simulink model "kinovaMicoSimscapeModel"  (R2021b)
settings: Solver=VariableStepAuto  StartTime=0.0  StopTime=0.3  FixedStep=0.01  RelTol=1e-3
PostLoadFcn:
  | micoRigidBodyTreeCreation;
  | IC=deg2rad([-90,180,180,0,0,0]);
  | interactiveHomePosition=deg2rad([-90 90 177.5 90 0 0]');
  | load("./KinovaMicoSimscapeVariantConfigurations.mat");
values from neighbouring files (symbols this model uses):
  micoCandlePosition = deg2rad([0,180,180,0,0,0])    [KinovaMicoSimscapeInitializeScript.m]    (also in generatingRandomTrajectory.m)
  ViaPointsTaskSpace = [ViaPointsTaskSpace;[[pi;0;pi],[pi;0;pi],[pi;0;pi],[pi;0;pi],[0;0;0],[0;0;0],[pi;0;pi]]]    [KinovaMicoSimscapeInitializeScript.m]    (also in generatingRandomTrajectory.m = [ViaPointsTaskSpace;zeros(3,7)])
undefined symbols (not defined in the file or in its folder): Mico, ViaPointsJointSpace, X, Y, Z
libraries: sm_lib x26, nesl_utility x19, robotcorelib x4, robotmaniplib x3, pid_lib x2
(part 1 of 50)
settings Model: VariantConfigurationObject=KinovaMicoSimscapeVariantConfigurations  Creator=Chris  LastModifiedBy=morle
settings SolverCC: AlgebraicLoopSolver=TrustRegion
settings DebuggingCC: SFMachineParentedDataDiag=warning

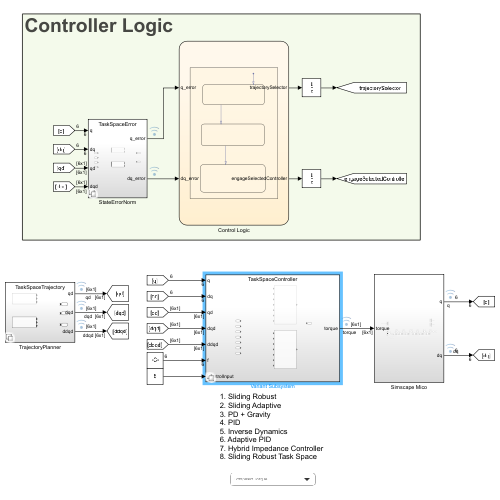
[thumbnail: Simulink's stored preview of the top-level diagram]
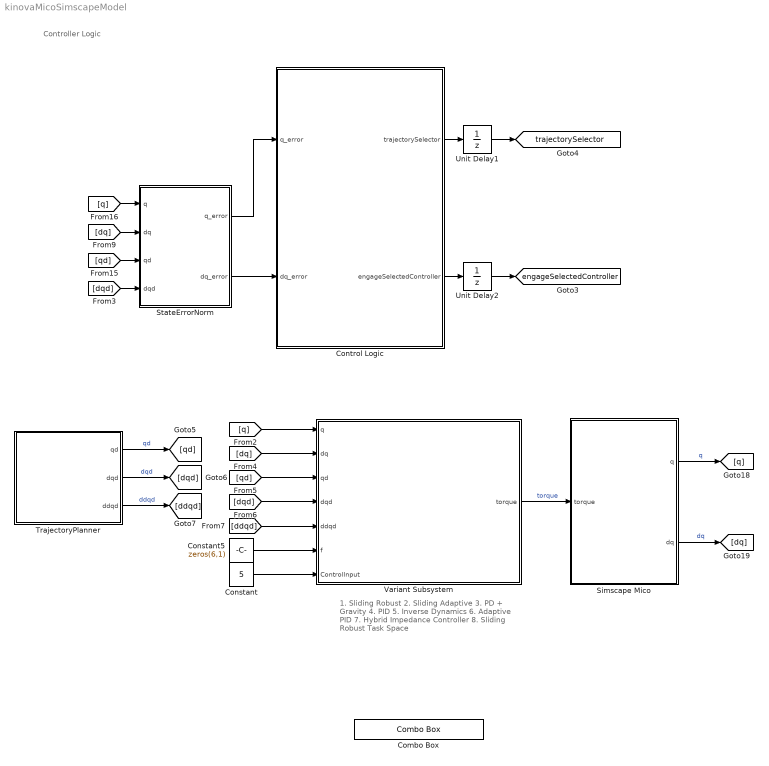
== system kinovaMicoSimscapeModel ==
  note: 1. Sliding Robust
      | 2. Sliding Adaptive
      | 3. PD + Gravity
      | 4. PID
      | 5. Inverse Dynamics
      | 6. Adaptive PID
      | 7. Hybrid Impedance Controller
      | 8. Sliding Robust Task Space
  note: Controller Logic
  Combo Box : ComboBox  LabelPosition=Hide  SelectedLabel=Computed Torque
      settings: Values={{'Sliding Robust Control', 'Sliding Adaptive Control', 'PD + Gravity', 'PID', 'Computed Torque', 'Adaptive PID', 'Hybrid Impedance Control', 'Sliding Robust Task Space'}, [1 2 3 4 5 6 7 8]}
  Constant : Constant  Value=5
  Constant5 : Constant  Value=zeros(6,1)
  Control Logic : Stateflow chart  TreatAsAtomicUnit=on
  Simscape Mico : Subsystem
  StateErrorNorm : Subsystem  Variant=on
  TrajectoryPlanner : Subsystem  Variant=on
  Unit Delay1 : UnitDelay  SampleTime=-1  HasFrameUpgradeWarning=on
  Unit Delay2 : UnitDelay  SampleTime=-1  HasFrameUpgradeWarning=on
  Variant Subsystem : Subsystem  Variant=on
  tag scope: engageSelectedController=global, trajectorySelector=global
  wires:
  Control Logic/2(engageSelectedController) -> Unit Delay2/1
  Unit Delay2/1 -> [engageSelectedController]
  Simscape Mico/2(dq) -> [dq]  "dq"
  Simscape Mico/1(q) -> [q]  "q"
  [dqd] -> Variant Subsystem/4(dqd)
  [ddqd] -> Variant Subsystem/5(ddqd)
  Constant5/1 -> Variant Subsystem/6(f)
  [dqd] -> StateErrorNorm/4(dqd)
  [dq] -> StateErrorNorm/2(dq)
  [qd] -> StateErrorNorm/3(qd)
  [q] -> StateErrorNorm/1(q)
  Variant Subsystem/1(torque) -> Simscape Mico/1(torque)  "torque"
  Unit Delay1/1 -> [trajectorySelector]
  Control Logic/1(trajectorySelector) -> Unit Delay1/1
  Constant/1 -> Variant Subsystem/7(ControlInput)
  [q] -> Variant Subsystem/1(q)
  [dq] -> Variant Subsystem/2(dq)
  [qd] -> Variant Subsystem/3(qd)
  StateErrorNorm/2(dq_error) -> Control Logic/2(dq_error)
  StateErrorNorm/1(q_error) -> Control Logic/1(q_error)
  TrajectoryPlanner/2(dqd) -> [dqd]  "dqd"
  TrajectoryPlanner/1(qd) -> [qd]  "qd"
  TrajectoryPlanner/3(ddqd) -> [ddqd]  "ddqd"

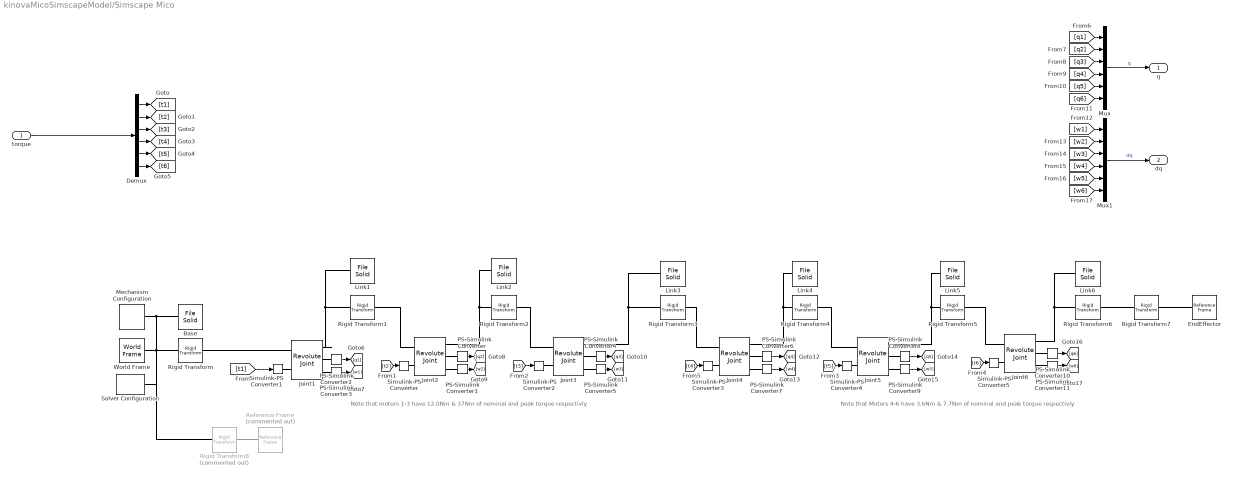
== system kinovaMicoSimscapeModel/Simscape Mico ==
  note: Note that motors 1-3 have 12.0Nm & 37Nm of nominal and peak torque respectivly
  note: Note that Motors 4-6 have 3.6Nm & 7.7Nm of nominal and peak torque respectivly
  torque : Inport
  Base : sm_lib/Body Elements/File Solid  ExtGeomFileName=.\StepFiles\Base.step  UnitType=FromFile  ExtGeomFileUnits=m  StepReaderType=HEX  ExportConvexHullGeometry=off  InertiaType=Custom  Mass=0  MassUnits=kg  CenterOfMass=[0 0 0]  CenterOfMassUnits=m  MomentsOfInertia=[0 0 0]  MomentsOfInertiaUnits=kg*m^2  ProductsOfInertia=[0 0 0]  ProductsOfInertiaUnits=kg*m^2  BasedOnType=Density  Density=1000  DensityUnits=kg/m^3  DoExposeReferenceFrame=on  SerializedFrames=<Frames/>  GraphicType=FromGeometry  MarkerShape=Sphere  MarkerSize=10  GraphicVisPropType=SimpleVisualProperties  GraphicDiffuseColor=[0.5 0.5 0.5]  GraphicSpecularColor=[0.5 0.5 0.5 1.0]  GraphicAmbientColor=[0.15 0.15 0.15 1.0]  GraphicEmissiveColor=[0.0 0.0 0.0 1.0]  GraphicShininess=75  GraphicOpacity=1.0
  Demux : Demux  Outputs=6
  EndEffector : sm_lib/Frames and Transforms/Reference Frame
  Joint1 : sm_lib/Joints/Revolute Joint  JointMode=Normal  SenseConstraintForce=off  SenseConstraintForceX=off  SenseConstraintForceY=off  SenseConstraintForceZ=off  SenseConstraintTorque=off  SenseConstraintTorqueX=off  SenseConstraintTorqueY=off  SenseConstraintTorqueZ=off  SenseTotalForce=off  SenseTotalForceX=off  SenseTotalForceY=off  SenseTotalForceZ=off  SenseTotalTorque=off  SenseTotalTorqueX=off  SenseTotalTorqueY=off  SenseTotalTorqueZ=off  CompositeWrenchDir=FollowerOnBase  CompositeWrenchFrame=BaseFrame  EquilibriumPosition=0  EquilibriumPositionUnits=deg  SpringStiffness=0  SpringStiffnessUnits=N*m/deg  DampingCoefficient=0.1  DampingCoefficientUnits=N*m/(deg/s)  TorqueActuationMode=InputTorque  MotionActuationMode=ComputedMotion  SensePosition=on  SenseVelocity=on  SenseAcceleration=off  SenseTorqueForce=off  SenseLowerLimitTorqueForce=off  SenseUpperLimitTorqueForce=off  LowerLimitSpecify=off  LowerLimitBound=-90  LowerLimitBoundUnits=deg  LowerLimitStiffness=1e4  LowerLimitStiffnessUnits=N*m/deg  LowerLimitDamping=10  LowerLimitDampingUnits=N*m/(deg/s)  LowerLimitTransitionRegionWidth=0.1  LowerLimitTransitionRegionWidthUnits=deg  UpperLimitSpecify=off  UpperLimitBound=90  UpperLimitBoundUnits=deg  UpperLimitStiffness=1e4  UpperLimitStiffnessUnits=N*m/deg  UpperLimitDamping=10  UpperLimitDampingUnits=N*m/(deg/s)  UpperLimitTransitionRegionWidth=0.1  UpperLimitTransitionRegionWidthUnits=deg  PositionTargetSpecify=on  PositionTargetPriority=High  PositionTargetValue=IC(1)  PositionTargetValueUnits=rad  VelocityTargetSpecify=off  VelocityTargetPriority=High  VelocityTargetValue=0  VelocityTargetValueUnits=deg/s
  Joint2 : sm_lib/Joints/Revolute Joint  JointMode=Normal  SenseConstraintForce=off  SenseConstraintForceX=off  SenseConstraintForceY=off  SenseConstraintForceZ=off  SenseConstraintTorque=off  SenseConstraintTorqueX=off  SenseConstraintTorqueY=off  SenseConstraintTorqueZ=off  SenseTotalForce=off  SenseTotalForceX=off  SenseTotalForceY=off  SenseTotalForceZ=off  SenseTotalTorque=off  SenseTotalTorqueX=off  SenseTotalTorqueY=off  SenseTotalTorqueZ=off  CompositeWrenchDir=FollowerOnBase  CompositeWrenchFrame=BaseFrame  EquilibriumPosition=0  EquilibriumPositionUnits=deg  SpringStiffness=0  SpringStiffnessUnits=N*m/deg  DampingCoefficient=.1  DampingCoefficientUnits=N*m/(deg/s)  TorqueActuationMode=InputTorque  MotionActuationMode=ComputedMotion  SensePosition=on  SenseVelocity=on  SenseAcceleration=off  SenseTorqueForce=off  SenseLowerLimitTorqueForce=off  SenseUpperLimitTorqueForce=off  LowerLimitSpecify=off  LowerLimitBound=-90  LowerLimitBoundUnits=deg  LowerLimitStiffness=1e4  LowerLimitStiffnessUnits=N*m/deg  LowerLimitDamping=10  LowerLimitDampingUnits=N*m/(deg/s)  LowerLimitTransitionRegionWidth=0.1  LowerLimitTransitionRegionWidthUnits=deg  UpperLimitSpecify=off  UpperLimitBound=90  UpperLimitBoundUnits=deg  UpperLimitStiffness=1e4  UpperLimitStiffnessUnits=N*m/deg  UpperLimitDamping=10  UpperLimitDampingUnits=N*m/(deg/s)  UpperLimitTransitionRegionWidth=0.1  UpperLimitTransitionRegionWidthUnits=deg  PositionTargetSpecify=on  PositionTargetPriority=High  PositionTargetValue=IC(2)  PositionTargetValueUnits=rad  VelocityTargetSpecify=off  VelocityTargetPriority=High  VelocityTargetValue=0  VelocityTargetValueUnits=deg/s
  Joint3 : sm_lib/Joints/Revolute Joint  JointMode=Normal  SenseConstraintForce=off  SenseConstraintForceX=off  SenseConstraintForceY=off  SenseConstraintForceZ=off  SenseConstraintTorque=off  SenseConstraintTorqueX=off  SenseConstraintTorqueY=off  SenseConstraintTorqueZ=off  SenseTotalForce=off  SenseTotalForceX=off  SenseTotalForceY=off  SenseTotalForceZ=off  SenseTotalTorque=off  SenseTotalTorqueX=off  SenseTotalTorqueY=off  SenseTotalTorqueZ=off  CompositeWrenchDir=FollowerOnBase  CompositeWrenchFrame=BaseFrame  EquilibriumPosition=0  EquilibriumPositionUnits=deg  SpringStiffness=0  SpringStiffnessUnits=N*m/deg  DampingCoefficient=.1  DampingCoefficientUnits=N*m/(deg/s)  TorqueActuationMode=InputTorque  MotionActuationMode=ComputedMotion  SensePosition=on  SenseVelocity=on  SenseAcceleration=off  SenseTorqueForce=off  SenseLowerLimitTorqueForce=off  SenseUpperLimitTorqueForce=off  LowerLimitSpecify=off  LowerLimitBound=-90  LowerLimitBoundUnits=deg  LowerLimitStiffness=1e4  LowerLimitStiffnessUnits=N*m/deg  LowerLimitDamping=10  LowerLimitDampingUnits=N*m/(deg/s)  LowerLimitTransitionRegionWidth=0.1  LowerLimitTransitionRegionWidthUnits=deg  UpperLimitSpecify=off  UpperLimitBound=90  UpperLimitBoundUnits=deg  UpperLimitStiffness=1e4  UpperLimitStiffnessUnits=N*m/deg  UpperLimitDamping=10  UpperLimitDampingUnits=N*m/(deg/s)  UpperLimitTransitionRegionWidth=0.1  UpperLimitTransitionRegionWidthUnits=deg  PositionTargetSpecify=on  PositionTargetPriority=High  PositionTargetValue=IC(3)  PositionTargetValueUnits=rad  VelocityTargetSpecify=off  VelocityTargetPriority=High  VelocityTargetValue=0  VelocityTargetValueUnits=deg/s
  Joint4 : sm_lib/Joints/Revolute Joint  JointMode=Normal  SenseConstraintForce=off  SenseConstraintForceX=off  SenseConstraintForceY=off  SenseConstraintForceZ=off  SenseConstraintTorque=off  SenseConstraintTorqueX=off  SenseConstraintTorqueY=off  SenseConstraintTorqueZ=off  SenseTotalForce=off  SenseTotalForceX=off  SenseTotalForceY=off  SenseTotalForceZ=off  SenseTotalTorque=off  SenseTotalTorqueX=off  SenseTotalTorqueY=off  SenseTotalTorqueZ=off  CompositeWrenchDir=FollowerOnBase  CompositeWrenchFrame=BaseFrame  EquilibriumPosition=0  EquilibriumPositionUnits=deg  SpringStiffness=0  SpringStiffnessUnits=N*m/deg  DampingCoefficient=.1  DampingCoefficientUnits=N*m/(deg/s)  TorqueActuationMode=InputTorque  MotionActuationMode=ComputedMotion  SensePosition=on  SenseVelocity=on  SenseAcceleration=off  SenseTorqueForce=off  SenseLowerLimitTorqueForce=off  SenseUpperLimitTorqueForce=off  LowerLimitSpecify=off  LowerLimitBound=-90  LowerLimitBoundUnits=deg  LowerLimitStiffness=1e4  LowerLimitStiffnessUnits=N*m/deg  LowerLimitDamping=10  LowerLimitDampingUnits=N*m/(deg/s)  LowerLimitTransitionRegionWidth=0.1  LowerLimitTransitionRegionWidthUnits=deg  UpperLimitSpecify=off  UpperLimitBound=90  UpperLimitBoundUnits=deg  UpperLimitStiffness=1e4  UpperLimitStiffnessUnits=N*m/deg  UpperLimitDamping=10  UpperLimitDampingUnits=N*m/(deg/s)  UpperLimitTransitionRegionWidth=0.1  UpperLimitTransitionRegionWidthUnits=deg  PositionTargetSpecify=on  PositionTargetPriority=High  PositionTargetValue=IC(4)  PositionTargetValueUnits=rad  VelocityTargetSpecify=off  VelocityTargetPriority=High  VelocityTargetValue=0  VelocityTargetValueUnits=deg/s
  Joint5 : sm_lib/Joints/Revolute Joint  JointMode=Normal  SenseConstraintForce=off  SenseConstraintForceX=off  SenseConstraintForceY=off  SenseConstraintForceZ=off  SenseConstraintTorque=off  SenseConstraintTorqueX=off  SenseConstraintTorqueY=off  SenseConstraintTorqueZ=off  SenseTotalForce=off  SenseTotalForceX=off  SenseTotalForceY=off  SenseTotalForceZ=off  SenseTotalTorque=off  SenseTotalTorqueX=off  SenseTotalTorqueY=off  SenseTotalTorqueZ=off  CompositeWrenchDir=FollowerOnBase  CompositeWrenchFrame=BaseFrame  EquilibriumPosition=0  EquilibriumPositionUnits=deg  SpringStiffness=0  SpringStiffnessUnits=N*m/deg  DampingCoefficient=.1  DampingCoefficientUnits=N*m/(deg/s)  TorqueActuationMode=InputTorque  MotionActuationMode=ComputedMotion  SensePosition=on  SenseVelocity=on  SenseAcceleration=off  SenseTorqueForce=off  SenseLowerLimitTorqueForce=off  SenseUpperLimitTorqueForce=off  LowerLimitSpecify=off  LowerLimitBound=-90  LowerLimitBoundUnits=deg  LowerLimitStiffness=1e4  LowerLimitStiffnessUnits=N*m/deg  LowerLimitDamping=10  LowerLimitDampingUnits=N*m/(deg/s)  LowerLimitTransitionRegionWidth=0.1  LowerLimitTransitionRegionWidthUnits=deg  UpperLimitSpecify=off  UpperLimitBound=90  UpperLimitBoundUnits=deg  UpperLimitStiffness=1e4  UpperLimitStiffnessUnits=N*m/deg  UpperLimitDamping=10  UpperLimitDampingUnits=N*m/(deg/s)  UpperLimitTransitionRegionWidth=0.1  UpperLimitTransitionRegionWidthUnits=deg  PositionTargetSpecify=on  PositionTargetPriority=High  PositionTargetValue=IC(5)  PositionTargetValueUnits=rad  VelocityTargetSpecify=off  VelocityTargetPriority=High  VelocityTargetValue=0  VelocityTargetValueUnits=deg/s
  Joint6 : sm_lib/Joints/Revolute Joint  JointMode=Normal  SenseConstraintForce=off  SenseConstraintForceX=off  SenseConstraintForceY=off  SenseConstraintForceZ=off  SenseConstraintTorque=off  SenseConstraintTorqueX=off  SenseConstraintTorqueY=off  SenseConstraintTorqueZ=off  SenseTotalForce=off  SenseTotalForceX=off  SenseTotalForceY=off  SenseTotalForceZ=off  SenseTotalTorque=off  SenseTotalTorqueX=off  SenseTotalTorqueY=off  SenseTotalTorqueZ=off  CompositeWrenchDir=FollowerOnBase  CompositeWrenchFrame=BaseFrame  EquilibriumPosition=0  EquilibriumPositionUnits=deg  SpringStiffness=0  SpringStiffnessUnits=N*m/deg  DampingCoefficient=.1  DampingCoefficientUnits=N*m/(deg/s)  TorqueActuationMode=InputTorque  MotionActuationMode=ComputedMotion  SensePosition=on  SenseVelocity=on  SenseAcceleration=off  SenseTorqueForce=off  SenseLowerLimitTorqueForce=off  SenseUpperLimitTorqueForce=off  LowerLimitSpecify=off  LowerLimitBound=-90  LowerLimitBoundUnits=deg  LowerLimitStiffness=1e4  LowerLimitStiffnessUnits=N*m/deg  LowerLimitDamping=10  LowerLimitDampingUnits=N*m/(deg/s)  LowerLimitTransitionRegionWidth=0.1  LowerLimitTransitionRegionWidthUnits=deg  UpperLimitSpecify=off  UpperLimitBound=90  UpperLimitBoundUnits=deg  UpperLimitStiffness=1e4  UpperLimitStiffnessUnits=N*m/deg  UpperLimitDamping=10  UpperLimitDampingUnits=N*m/(deg/s)  UpperLimitTransitionRegionWidth=0.1  UpperLimitTransitionRegionWidthUnits=deg  PositionTargetSpecify=on  PositionTargetPriority=High  PositionTargetValue=IC(6)  PositionTargetValueUnits=rad  VelocityTargetSpecify=off  VelocityTargetPriority=High  VelocityTargetValue=0  VelocityTargetValueUnits=deg/s
  Link1 : sm_lib/Body Elements/File Solid  ExtGeomFileName=.\StepFiles\Link1.step  UnitType=FromFile  ExtGeomFileUnits=m  StepReaderType=HEX  ExportConvexHullGeometry=off  InertiaType=Custom  Mass=Mico.Mass{1}  MassUnits=kg  CenterOfMass=Mico.COM{1}  CenterOfMassUnits=m  MomentsOfInertia=Mico.Inertia{1}(1:3)  MomentsOfInertiaUnits=kg*m^2  ProductsOfInertia=Mico.Inertia{1}(4:6)  ProductsOfInertiaUnits=kg*m^2  BasedOnType=Density  Density=1000  DensityUnits=kg/m^3  DoExposeReferenceFrame=on  SerializedFrames=<Frames/>  GraphicType=FromGeometry  MarkerShape=Sphere  MarkerSize=10  GraphicVisPropType=SimpleVisualProperties  GraphicDiffuseColor=[0.5 0.5 0.5]  GraphicSpecularColor=[0.5 0.5 0.5 1.0]  GraphicAmbientColor=[0.15 0.15 0.15 1.0]  GraphicEmissiveColor=[0.0 0.0 0.0 1.0]  GraphicShininess=75  GraphicOpacity=1.0
  Link2 : sm_lib/Body Elements/File Solid  ExtGeomFileName=.\StepFiles\Link2.step  UnitType=FromFile  ExtGeomFileUnits=m  StepReaderType=HEX  ExportConvexHullGeometry=off  InertiaType=Custom  Mass=Mico.Mass{2}  MassUnits=kg  CenterOfMass=Mico.COM{2}  CenterOfMassUnits=m  MomentsOfInertia=Mico.Inertia{2}(1:3)  MomentsOfInertiaUnits=kg*m^2  ProductsOfInertia=Mico.Inertia{2}(4:6)  ProductsOfInertiaUnits=kg*m^2  BasedOnType=Density  Density=1000  DensityUnits=kg/m^3  DoExposeReferenceFrame=on  SerializedFrames=<Frames/>  GraphicType=FromGeometry  MarkerShape=Sphere  MarkerSize=10  GraphicVisPropType=SimpleVisualProperties  GraphicDiffuseColor=[0.5 0.5 0.5]  GraphicSpecularColor=[0.5 0.5 0.5 1.0]  GraphicAmbientColor=[0.15 0.15 0.15 1.0]  GraphicEmissiveColor=[0.0 0.0 0.0 1.0]  GraphicShininess=75  GraphicOpacity=1.0
  Link3 : sm_lib/Body Elements/File Solid  ExtGeomFileName=.\StepFiles\Link3.step  UnitType=FromFile  ExtGeomFileUnits=m  StepReaderType=HEX  ExportConvexHullGeometry=off  InertiaType=Custom  Mass=Mico.Mass{3}  MassUnits=kg  CenterOfMass=Mico.COM{3}  CenterOfMassUnits=m  MomentsOfInertia=Mico.Inertia{3}(1:3)  MomentsOfInertiaUnits=kg*m^2  ProductsOfInertia=Mico.Inertia{3}(4:6)  ProductsOfInertiaUnits=kg*m^2  BasedOnType=Density  Density=1000  DensityUnits=kg/m^3  DoExposeReferenceFrame=on  SerializedFrames=<Frames/>  GraphicType=FromGeometry  MarkerShape=Sphere  MarkerSize=10  GraphicVisPropType=SimpleVisualProperties  GraphicDiffuseColor=[0.5 0.5 0.5]  GraphicSpecularColor=[0.5 0.5 0.5 1.0]  GraphicAmbientColor=[0.15 0.15 0.15 1.0]  GraphicEmissiveColor=[0.0 0.0 0.0 1.0]  GraphicShininess=75  GraphicOpacity=1.0
  Link4 : sm_lib/Body Elements/File Solid  ExtGeomFileName=.\StepFiles\Link4.step  UnitType=FromFile  ExtGeomFileUnits=m  StepReaderType=HEX  ExportConvexHullGeometry=off  InertiaType=Custom  Mass=Mico.Mass{4}  MassUnits=kg  CenterOfMass=Mico.COM{4}  CenterOfMassUnits=m  MomentsOfInertia=Mico.Inertia{4}(1:3)  MomentsOfInertiaUnits=kg*m^2  ProductsOfInertia=Mico.Inertia{4}(4:6)  ProductsOfInertiaUnits=kg*m^2  BasedOnType=Density  Density=1000  DensityUnits=kg/m^3  DoExposeReferenceFrame=on  SerializedFrames=<Frames/>  GraphicType=FromGeometry  MarkerShape=Sphere  MarkerSize=10  GraphicVisPropType=SimpleVisualProperties  GraphicDiffuseColor=[0.5 0.5 0.5]  GraphicSpecularColor=[0.5 0.5 0.5 1.0]  GraphicAmbientColor=[0.15 0.15 0.15 1.0]  GraphicEmissiveColor=[0.0 0.0 0.0 1.0]  GraphicShininess=75  GraphicOpacity=1.0
  Link5 : sm_lib/Body Elements/File Solid  ExtGeomFileName=.\StepFiles\Link5.step  UnitType=FromFile  ExtGeomFileUnits=m  StepReaderType=HEX  ExportConvexHullGeometry=off  InertiaType=Custom  Mass=Mico.Mass{5}  MassUnits=kg  CenterOfMass=Mico.COM{5}  CenterOfMassUnits=m  MomentsOfInertia=Mico.Inertia{5}(1:3)  MomentsOfInertiaUnits=kg*m^2  ProductsOfInertia=Mico.Inertia{5}(4:6)  ProductsOfInertiaUnits=kg*m^2  BasedOnType=Density  Density=1000  DensityUnits=kg/m^3  DoExposeReferenceFrame=on  SerializedFrames=<Frames/>  GraphicType=FromGeometry  MarkerShape=Sphere  MarkerSize=10  GraphicVisPropType=SimpleVisualProperties  GraphicDiffuseColor=[0.5 0.5 0.5]  GraphicSpecularColor=[0.5 0.5 0.5 1.0]  GraphicAmbientColor=[0.15 0.15 0.15 1.0]  GraphicEmissiveColor=[0.0 0.0 0.0 1.0]  GraphicShininess=75  GraphicOpacity=1.0
  Link6 : sm_lib/Body Elements/File Solid  ExtGeomFileName=.\StepFiles\forceSensorEE.stl  UnitType=Custom  ExtGeomFileUnits=m  StepReaderType=HEX  ExportConvexHullGeometry=off  InertiaType=Custom  Mass=Mico.Mass{6}  MassUnits=kg  CenterOfMass=Mico.COM{6}  CenterOfMassUnits=m  MomentsOfInertia=Mico.Inertia{6}(1:3)  MomentsOfInertiaUnits=kg*m^2  ProductsOfInertia=Mico.Inertia{6}(4:6)  ProductsOfInertiaUnits=kg*m^2  BasedOnType=Density  Density=1000  DensityUnits=kg/m^3  DoExposeReferenceFrame=on  SerializedFrames=<Frames/>  GraphicType=FromGeometry  MarkerShape=Sphere  MarkerSize=10  GraphicVisPropType=SimpleVisualProperties  GraphicDiffuseColor=[0.5 0.5 0.5]  GraphicSpecularColor=[0.5 0.5 0.5 1.0]  GraphicAmbientColor=[0.15 0.15 0.15 1.0]  GraphicEmissiveColor=[0.0 0.0 0.0 1.0]  GraphicShininess=75  GraphicOpacity=1.0
  Mechanism Configuration : sm_lib/Utilities/Mechanism Configuration  UniformGravity=Constant  GravityVector=[0 0 -9.81]  GravityUnits=m/s^2  LinearizationDelta=0.001  JointModeTransitionNonlinearIterations=2
  Mux : Mux  Inputs=6
  Mux1 : Mux  Inputs=6
  PS-Simulink Converter{,1..11} (12 alike) : nesl_utility/PS-Simulink Converter  PhysicalDomain=network_engine_domain  SubClassName=ps_output  LeftPortType=input  RightPortType=output  PseudoPeriodic=off  Frequencies=[]  Unit=inherit  AffineConversion=off
      settings: SourceProductBaseCode=PW,SS
  Reference Frame : sm_lib/Frames and Transforms/Reference Frame  Commented=on
  Rigid Transform : sm_lib/Frames and Transforms/Rigid Transform  TranslationMethod=Cartesian  TranslationStandardOffset=0  TranslationLengthUnit=m  TranslationStandardAxis=+Z  TranslationCartesianOffset=Mico.JointTransforms.Translation{1}  TranslationROffset=0  TranslationROffsetUnits=m  TranslationZOffset=0  TranslationZOffsetUnits=m  TranslationThetaOffset=0  TranslationThetaOffsetUnits=deg  RotationMethod=RotationMatrix  RotationAngleUnits=deg  RotationStandardAxis=+Z  RotationAngle=0.0  RotationArbitraryAxis=[0 0 1]  FollAlignAxisA=+X  BaseAlignAxisA=+Y  FollAlignAxisB=+Y  BaseAlignAxisB=+Z  RotationSequenceAxes=FollowerAxes  RotationSequence=XYX  RotationSequenceAngles=[0 0 0]  RotationSequenceAnglesUnits=deg  RotationMatrix=Mico.JointTransforms.Rotation{1}
  Rigid Transform1 : sm_lib/Frames and Transforms/Rigid Transform  TranslationMethod=Cartesian  TranslationStandardOffset=0  TranslationLengthUnit=m  TranslationStandardAxis=+Z  TranslationCartesianOffset=Mico.JointTransforms.Translation{2}  TranslationROffset=0  TranslationROffsetUnits=m  TranslationZOffset=0  TranslationZOffsetUnits=m  TranslationThetaOffset=0  TranslationThetaOffsetUnits=deg  RotationMethod=RotationMatrix  RotationAngleUnits=deg  RotationStandardAxis=+Z  RotationAngle=0.0  RotationArbitraryAxis=[0 0 1]  FollAlignAxisA=+X  BaseAlignAxisA=+Y  FollAlignAxisB=+Y  BaseAlignAxisB=+Z  RotationSequenceAxes=FollowerAxes  RotationSequence=XYX  RotationSequenceAngles=[0 0 0]  RotationSequenceAnglesUnits=deg  RotationMatrix=Mico.JointTransforms.Rotation{2}
  Rigid Transform2 : sm_lib/Frames and Transforms/Rigid Transform  TranslationMethod=Cartesian  TranslationStandardOffset=0  TranslationLengthUnit=m  TranslationStandardAxis=+Z  TranslationCartesianOffset=Mico.JointTransforms.Translation{3}  TranslationROffset=0  TranslationROffsetUnits=m  TranslationZOffset=0  TranslationZOffsetUnits=m  TranslationThetaOffset=0  TranslationThetaOffsetUnits=deg  RotationMethod=RotationMatrix  RotationAngleUnits=deg  RotationStandardAxis=+Z  RotationAngle=0.0  RotationArbitraryAxis=[0 0 1]  FollAlignAxisA=+X  BaseAlignAxisA=+Y  FollAlignAxisB=+Y  BaseAlignAxisB=+Z  RotationSequenceAxes=FollowerAxes  RotationSequence=XYX  RotationSequenceAngles=[0 0 0]  RotationSequenceAnglesUnits=deg  RotationMatrix=Mico.JointTransforms.Rotation{3}
  Rigid Transform3 : sm_lib/Frames and Transforms/Rigid Transform  TranslationMethod=Cartesian  TranslationStandardOffset=0  TranslationLengthUnit=m  TranslationStandardAxis=+Z  TranslationCartesianOffset=Mico.JointTransforms.Translation{4}  TranslationROffset=0  TranslationROffsetUnits=m  TranslationZOffset=0  TranslationZOffsetUnits=m  TranslationThetaOffset=0  TranslationThetaOffsetUnits=deg  RotationMethod=RotationMatrix  RotationAngleUnits=deg  RotationStandardAxis=+Z  RotationAngle=0.0  RotationArbitraryAxis=[0 0 1]  FollAlignAxisA=+X  BaseAlignAxisA=+Y  FollAlignAxisB=+Y  BaseAlignAxisB=+Z  RotationSequenceAxes=FollowerAxes  RotationSequence=XYX  RotationSequenceAngles=[0 0 0]  RotationSequenceAnglesUnits=deg  RotationMatrix=Mico.JointTransforms.Rotation{4}
  Rigid Transform4 : sm_lib/Frames and Transforms/Rigid Transform  TranslationMethod=Cartesian  TranslationStandardOffset=0  TranslationLengthUnit=m  TranslationStandardAxis=+Z  TranslationCartesianOffset=Mico.JointTransforms.Translation{5}  TranslationROffset=0  TranslationROffsetUnits=m  TranslationZOffset=0  TranslationZOffsetUnits=m  TranslationThetaOffset=0  TranslationThetaOffsetUnits=deg  RotationMethod=RotationMatrix  RotationAngleUnits=deg  RotationStandardAxis=+Z  RotationAngle=0.0  RotationArbitraryAxis=[0 0 1]  FollAlignAxisA=+X  BaseAlignAxisA=+Y  FollAlignAxisB=+Y  BaseAlignAxisB=+Z  RotationSequenceAxes=FollowerAxes  RotationSequence=XYX  RotationSequenceAngles=[0 0 0]  RotationSequenceAnglesUnits=deg  RotationMatrix=Mico.JointTransforms.Rotation{5}
  Rigid Transform5 : sm_lib/Frames and Transforms/Rigid Transform  TranslationMethod=Cartesian  TranslationStandardOffset=0  TranslationLengthUnit=m  TranslationStandardAxis=+Z  TranslationCartesianOffset=Mico.JointTransforms.Translation{6}  TranslationROffset=0  TranslationROffsetUnits=m  TranslationZOffset=0  TranslationZOffsetUnits=m  TranslationThetaOffset=0  TranslationThetaOffsetUnits=deg  RotationMethod=RotationMatrix  RotationAngleUnits=deg  RotationStandardAxis=+Z  RotationAngle=0.0  RotationArbitraryAxis=[0 0 1]  FollAlignAxisA=+X  BaseAlignAxisA=+Y  FollAlignAxisB=+Y  BaseAlignAxisB=+Z  RotationSequenceAxes=FollowerAxes  RotationSequence=XYX  RotationSequenceAngles=[0 0 0]  RotationSequenceAnglesUnits=deg  RotationMatrix=Mico.JointTransforms.Rotation{6}
  Rigid Transform6 : sm_lib/Frames and Transforms/Rigid Transform  TranslationMethod=StandardAxis  TranslationStandardOffset=.123724  TranslationLengthUnit=m  TranslationStandardAxis=-Z  TranslationCartesianOffset=[0 0 0]  TranslationROffset=0  TranslationROffsetUnits=m  TranslationZOffset=0  TranslationZOffsetUnits=m  TranslationThetaOffset=0  TranslationThetaOffsetUnits=deg  RotationMethod=None  RotationAngleUnits=deg  RotationStandardAxis=+Z  RotationAngle=0.0  RotationArbitraryAxis=[0 0 1]  FollAlignAxisA=+X  BaseAlignAxisA=+Y  FollAlignAxisB=+Y  BaseAlignAxisB=+Z  RotationSequenceAxes=FollowerAxes  RotationSequence=XYX  RotationSequenceAngles=[0 0 0]  RotationSequenceAnglesUnits=deg  RotationMatrix=[1 0 0; 0 1 0; 0 0 1]
  Rigid Transform7 : sm_lib/Frames and Transforms/Rigid Transform  TranslationMethod=None  TranslationStandardOffset=.123724  TranslationLengthUnit=m  TranslationStandardAxis=-Z  TranslationCartesianOffset=[0 0 0]  TranslationROffset=0  TranslationROffsetUnits=m  TranslationZOffset=0  TranslationZOffsetUnits=m  TranslationThetaOffset=0  TranslationThetaOffsetUnits=deg  RotationMethod=StandardAxis  RotationAngleUnits=deg  RotationStandardAxis=+Y  RotationAngle=180  RotationArbitraryAxis=[0 0 1]  FollAlignAxisA=+X  BaseAlignAxisA=+Y  FollAlignAxisB=+Y  BaseAlignAxisB=+Z  RotationSequenceAxes=FollowerAxes  RotationSequence=XYX  RotationSequenceAngles=[0 0 0]  RotationSequenceAnglesUnits=deg  RotationMatrix=[1 0 0; 0 1 0; 0 0 1]
  Rigid Transform8 : sm_lib/Frames and Transforms/Rigid Transform  Commented=on  TranslationMethod=Cartesian  TranslationStandardOffset=0  TranslationLengthUnit=m  TranslationStandardAxis=+Z  TranslationCartesianOffset=ViaPointsTaskSpace(1:3,1)  TranslationROffset=0  TranslationROffsetUnits=m  TranslationZOffset=0  TranslationZOffsetUnits=m  TranslationThetaOffset=0  TranslationThetaOffsetUnits=deg  RotationMethod=RotationSequence  RotationAngleUnits=deg  RotationStandardAxis=+Z  RotationAngle=0.0  RotationArbitraryAxis=[0 0 1]  FollAlignAxisA=+X  BaseAlignAxisA=+Y  FollAlignAxisB=+Y  BaseAlignAxisB=+Z  RotationSequenceAxes=FollowerAxes  RotationSequence=XYZ  RotationSequenceAngles=[pi,0,pi]  RotationSequenceAnglesUnits=rad  RotationMatrix=[1 0 0; 0 1 0; 0 0 1]
  Simulink-PS Converter{,1..5} (6 alike) : nesl_utility/Simulink-PS Converter  PhysicalDomain=network_engine_domain  SubClassName=ps_input  LeftPortType=input  RightPortType=output  PseudoPeriodic=off  Frequencies=[]  NoiseDistribution=none  NoiseParameters=[]  Unit=1  AffineConversion=off  FilteringAndDerivatives=provide  SimscapeFilterOrder=1  InputFilterTimeConstant=0.001  UdotUserProvided=0
      settings: SourceProductBaseCode=PW,SS
  Solver Configuration : nesl_utility/Solver Configuration  PhysicalDomain=network_engine_domain  SubClassName=solver  LeftPortType=input  RightPortType=generic  Tones=[]  Harmonics=[]  SimulateNoise=off  Profile=off  UseLocalSampling=off  EnableSwitchedLinearOptims=on  FrequencyDomain=off  UseCCode=off  RelTol=0.001  AbsTol=1e-06  MinStep=1e-09  ToWorkspace=off  RevertToSquareIcSolve=off  NumHomotopyIterations=100  PhasorMode=off  PhasorModeNumHarmonics=1  DoDC=off  ResidualTolerance=1e-09  UseLocalSolver=off  LocalSolverChoice=NE_BACKWARD_EULER_ADVANCER  LocalSolverSampleTime=0.001  DoFixedCost=off  MaxNonlinIter=3  MaxModeIter=2  ComputeImpulses=off  ImpulseIterations=2  LinearAlgebra=auto  EquationFormulation=NE_TIME_EF  DelaysMemoryBudget=1024  AutomaticFiltering=on  FilteringTimeConstant=0.001  PartitionStorageMethod=AS_NEEDED  PartitionMemoryBudget=1024  PartitionMethod=ROBUST
      settings: SourceProductBaseCode=PW,SS
  World Frame : sm_lib/Frames and Transforms/World Frame
  q : Outport
  dq : Outport  Port=2
  wires:
  PS-Simulink Converter4/1 -> [q3]
  Demux/5 -> [t5]
  PS-Simulink Converter/1 -> [q2]
  [q5] -> Mux/5
  PS-Simulink Converter3/1 -> [w1]
  [w3] -> Mux1/3
  [t2] -> Simulink-PS Converter/1
  PS-Simulink Converter9/1 -> [w5]
  Demux/2 -> [t2]
  [t4] -> Simulink-PS Converter3/1
  Demux/6 -> [t6]
  [w6] -> Mux1/6
  [q2] -> Mux/2
  Demux/4 -> [t4]
  [w1] -> Mux1/1
  [t5] -> Simulink-PS Converter4/1
  [w5] -> Mux1/5
  PS-Simulink Converter10/1 -> [q6]
  [t3] -> Simulink-PS Converter2/1
  [q6] -> Mux/6
  PS-Simulink Converter5/1 -> [w3]
  [w4] -> Mux1/4
  [w2] -> Mux1/2
  PS-Simulink Converter6/1 -> [q4]
  [t1] -> Simulink-PS Converter1/1
  [t6] -> Simulink-PS Converter5/1
  PS-Simulink Converter7/1 -> [w4]
  [q1] -> Mux/1
  PS-Simulink Converter8/1 -> [q5]
  [q3] -> Mux/3
  PS-Simulink Converter1/1 -> [w2]
  Demux/1 -> [t1]
  Demux/3 -> [t3]
  [q4] -> Mux/4
  PS-Simulink Converter11/1 -> [w6]
  PS-Simulink Converter2/1 -> [q1]
  Mux/1 -> q/1  "q"
  Mux1/1 -> dq/1  "dq"
  torque/1 -> Demux/1
  connections:
  Joint5/RConn3 -- PS-Simulink Converter9/LConn1
  Link6/RConn1 -- Joint6/RConn1 -- Rigid Transform6/LConn1
  Link2/RConn1 -- Joint2/RConn1 -- Rigid Transform2/LConn1
  Link3/RConn1 -- Rigid Transform3/LConn1 -- Joint3/RConn1
  Joint1/LConn1 -- Rigid Transform/RConn1
  Joint6/LConn1 -- Rigid Transform5/RConn1
  Joint6/RConn3 -- PS-Simulink Converter11/LConn1
  Joint1/RConn3 -- PS-Simulink Converter3/LConn1
  Simulink-PS Converter1/RConn1 -- Joint1/LConn2
  Joint2/RConn3 -- PS-Simulink Converter1/LConn1
  PS-Simulink Converter/LConn1 -- Joint2/RConn2
  PS-Simulink Converter4/LConn1 -- Joint3/RConn2
  Rigid Transform2/RConn1 -- Joint3/LConn1
  PS-Simulink Converter6/LConn1 -- Joint4/RConn2
  Rigid Transform5/LConn1 -- Link5/RConn1 -- Joint5/RConn1
  PS-Simulink Converter8/LConn1 -- Joint5/RConn2
  Simulink-PS Converter3/RConn1 -- Joint4/LConn2
  Simulink-PS Converter2/RConn1 -- Joint3/LConn2
  Joint3/RConn3 -- PS-Simulink Converter5/LConn1
  Joint5/LConn1 -- Rigid Transform4/RConn1
  Rigid Transform3/RConn1 -- Joint4/LConn1
  Mechanism Configuration/RConn1 -- Rigid Transform8/LConn1 -- Solver Configuration/RConn1 -- Rigid Transform/LConn1 -- World Frame/RConn1 -- Base/RConn1
  PS-Simulink Converter10/LConn1 -- Joint6/RConn2
  Joint2/LConn1 -- Rigid Transform1/RConn1
  Rigid Transform4/LConn1 -- Joint4/RConn1 -- Link4/RConn1
  Rigid Transform1/LConn1 -- Link1/RConn1 -- Joint1/RConn1
  Joint4/RConn3 -- PS-Simulink Converter7/LConn1
  Simulink-PS Converter4/RConn1 -- Joint5/LConn2
  Simulink-PS Converter5/RConn1 -- Joint6/LConn2
  Simulink-PS Converter/RConn1 -- Joint2/LConn2
  PS-Simulink Converter2/LConn1 -- Joint1/RConn2
  Rigid Transform7/LConn1 -- Rigid Transform6/RConn1
  Rigid Transform7/RConn1 -- EndEffector/RConn1
  Reference Frame/RConn1 -- Rigid Transform8/RConn1

== system kinovaMicoSimscapeModel/StateErrorNorm ==
  q : Inport
  dq : Inport  Port=2
  qd : Inport  Port=3
  dqd : Inport  Port=4
  JointSpaceError : Subsystem  VariantControl=JointSpace
  TaskSpaceError : Subsystem  VariantControl=TaskSpace
  q_error : Outport
  dq_error : Outport  Port=2

== system kinovaMicoSimscapeModel/TrajectoryPlanner ==
  JointSpaceTrajectory : Subsystem  VariantControl=JointSpace
  TaskSpaceTrajectory : Subsystem  VariantControl=TaskSpace
  qd : Outport
  dqd : Outport  Port=2
  ddqd : Outport  Port=3

== system kinovaMicoSimscapeModel/Variant Subsystem ==
  q : Inport
  dq : Inport  Port=2
  qd : Inport  Port=3
  dqd : Inport  Port=4
  ddqd : Inport  Port=5
  f : Inport  Port=6
  ControlInput : Inport  Port=7
  JointSpaceController : Subsystem  VariantControl=JointSpace
  TaskSpaceController : Subsystem  VariantControl=TaskSpace
  torque : Outport

== system kinovaMicoSimscapeModel/StateErrorNorm/JointSpaceError ==
  q : Inport
  dq : Inport  Port=2
  qd : Inport  Port=3
  dqd : Inport  Port=4
  Compute dqError : Subsystem
  Compute qError : Subsystem
  q_error : Outport
  dq_error : Outport  Port=2
  wires:
  qd/1 -> Compute qError/2(q)
  dqd/1 -> Compute dqError/1(dqd)
  dq/1 -> Compute dqError/2(dq)
  q/1 -> Compute qError/1(qd)
  Compute dqError/1(dq_error) -> dq_error/1
  Compute qError/1(q_error) -> q_error/1

== system kinovaMicoSimscapeModel/StateErrorNorm/TaskSpaceError ==
  q : Inport
  dq : Inport  Port=2
  qd : Inport  Port=3
  dqd : Inport  Port=4
  Compute dqError : Subsystem
  Compute qError : Subsystem
  Coordinate Transformation Conversion : robotcorelib/Coordinate Transformation Conversion  InputRepresentation=Rotation Matrix  InputEulerSequence=ZYX  ShowTrVecInputPort=on  OutputRepresentation=Euler Angles  OutputEulerSequence=XYZ  ShowTrVecOutputPort=on  SimulateUsing=Code generation
      settings: SourceProductBaseCode=NV,RO,RR,UV
  Get Transform : robotmaniplib/Get Transform  RigidBodyTree=mico  SourceBody=EE  TargetBody=base  SimulateUsing=Code generation
  Matrix Multiply : Product  Multiplication=Matrix(*)
  MicoJac : MATLAB Function  TreatAsAtomicUnit=on
  Selector : Selector  NumberOfDimensions=2  InputPortWidth=3  IndexOptions=Index vector (dialog),Index vector (dialog)  Indices=[1:3],4  OutputSizes=1,1
  Selector1 : Selector  NumberOfDimensions=2  InputPortWidth=3  IndexOptions=Index vector (dialog),Index vector (dialog)  Indices=[1:3],[1:3]  OutputSizes=1,1
  Vector Concatenate : Concatenate
  q_error : Outport
  dq_error : Outport  Port=2
  wires:
  q/1 -> MicoJac/1(q), Get Transform/1
  Get Transform/1 -> Selector1/1, Selector/1
  qd/1 -> Compute qError/1(qd)
  dqd/1 -> Compute dqError/1(dqd)
  MicoJac/1(Jac) -> Matrix Multiply/1
  dq/1 -> Matrix Multiply/2
  Matrix Multiply/1 -> Compute dqError/2(dq)
  Compute qError/1(q_error) -> q_error/1
  Compute dqError/1(dq_error) -> dq_error/1
  Selector1/1 -> Coordinate Transformation Conversion/1
  Vector Concatenate/1 -> Compute qError/2(q)
  Selector/1 -> Vector Concatenate/1
  Coordinate Transformation Conversion/1 -> Vector Concatenate/2

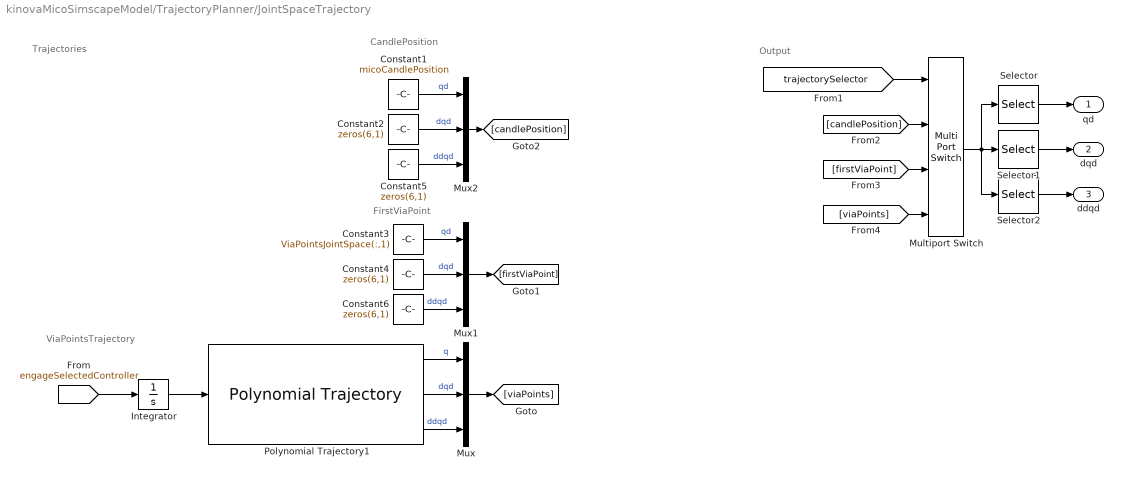
== system kinovaMicoSimscapeModel/TrajectoryPlanner/JointSpaceTrajectory ==
  note: Trajectories
  note: ViaPointsTrajectory
  note: FirstViaPoint
  note: CandlePosition
  note: Output
  Constant1 : Constant  Value=micoCandlePosition
  Constant{2,4..6} (4 alike) : Constant  Value=zeros(6,1)
  Constant3 : Constant  Value=ViaPointsJointSpace(:,1)
  Integrator : Integrator
  Multiport Switch : MultiPortSwitch  DataPortOrder=Zero-based contiguous  zeroidx=on
  Mux : Mux  Inputs=3
  Mux1 : Mux  Inputs=3
  Mux2 : Mux  Inputs=3
  Polynomial Trajectory1 : robotcorelib/Polynomial Trajectory  WaypointSource=Internal  Waypoints=ViaPointsJointSpace  TimePoints=t  TimeInterval=[ 1, 4 ]  Method=Cubic Polynomial  ParameterSource=Internal  VelocityBoundaryCondition=zeros(6,size(ViaPointsJointSpace,2))  AccelerationBoundaryCondition=zeros( 2, 5 )  SimulateUsing=Code generation
  Selector : Selector  InputPortWidth=18  IndexOptions=Index vector (dialog)  Indices=[1:6]  OutputSizes=1
  Selector1 : Selector  InputPortWidth=18  IndexOptions=Index vector (dialog)  Indices=[7:12]  OutputSizes=1
  Selector2 : Selector  InputPortWidth=18  IndexOptions=Index vector (dialog)  Indices=[13:18]  OutputSizes=1
  qd : Outport
  dqd : Outport  Port=2
  ddqd : Outport  Port=3
  wires:
  Constant3/1 -> Mux1/1  "qd"
  Selector2/1 -> ddqd/1
  Selector1/1 -> dqd/1
  Selector/1 -> qd/1
  Multiport Switch/1 -> Selector2/1, Selector/1, Selector1/1
  Mux/1 -> [viaPoints]
  Constant6/1 -> Mux1/3  "ddqd"
  Constant5/1 -> Mux2/3  "ddqd"
  [viaPoints] -> Multiport Switch/4
  [firstViaPoint] -> Multiport Switch/3
  [candlePosition] -> Multiport Switch/2
  Mux2/1 -> [candlePosition]
  Mux1/1 -> [firstViaPoint]
  Constant4/1 -> Mux1/2  "dqd"
  Constant2/1 -> Mux2/2  "dqd"
  Polynomial Trajectory1/2 -> Mux/2  "dqd"
  Polynomial Trajectory1/3 -> Mux/3  "ddqd"
  Polynomial Trajectory1/1 -> Mux/1  "q"
  [trajectorySelector] -> Multiport Switch/1
  Integrator/1 -> Polynomial Trajectory1/1
  [engageSelectedController] -> Integrator/1
  Constant1/1 -> Mux2/1  "qd"

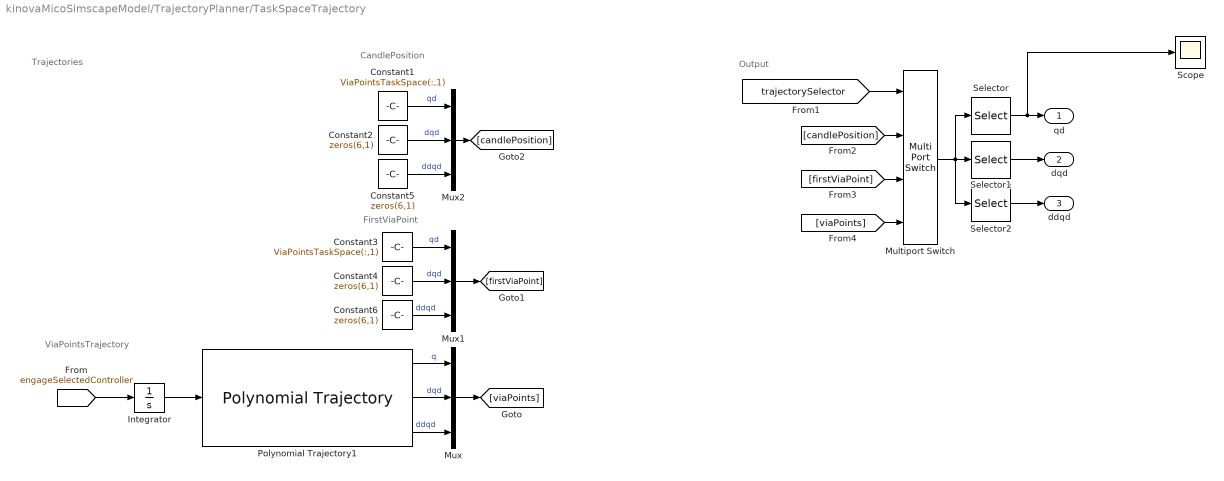
== system kinovaMicoSimscapeModel/TrajectoryPlanner/TaskSpaceTrajectory ==
  note: FirstViaPoint
  note: CandlePosition
  note: Trajectories
  note: ViaPointsTrajectory
  note: Output
  Constant1 : Constant  Value=ViaPointsTaskSpace(:,1)
  Constant{2,4..6} (4 alike) : Constant  Value=zeros(6,1)
  Constant3 : Constant  Value=ViaPointsTaskSpace(:,1)
  Integrator : Integrator
  Multiport Switch : MultiPortSwitch  DataPortOrder=Zero-based contiguous  zeroidx=on
  Mux : Mux  Inputs=3
  Mux1 : Mux  Inputs=3
  Mux2 : Mux  Inputs=3
  Polynomial Trajectory1 : robotcorelib/Polynomial Trajectory  WaypointSource=Internal  Waypoints=ViaPointsTaskSpace  TimePoints=t  TimeInterval=[ 1, 4 ]  Method=Cubic Polynomial  ParameterSource=Internal  VelocityBoundaryCondition=zeros(6,7)  AccelerationBoundaryCondition=zeros( 2, 5 )  SimulateUsing=Code generation
  Scope : Scope
  Selector : Selector  InputPortWidth=18  IndexOptions=Index vector (dialog)  Indices=[1:6]  OutputSizes=1
  Selector1 : Selector  InputPortWidth=18  IndexOptions=Index vector (dialog)  Indices=[7:12]  OutputSizes=1
  Selector2 : Selector  InputPortWidth=18  IndexOptions=Index vector (dialog)  Indices=[13:18]  OutputSizes=1
  qd : Outport
  dqd : Outport  Port=2
  ddqd : Outport  Port=3
  wires:
  Constant1/1 -> Mux2/1  "qd"
  [trajectorySelector] -> Multiport Switch/1
  Polynomial Trajectory1/1 -> Mux/1  "q"
  Integrator/1 -> Polynomial Trajectory1/1
  Polynomial Trajectory1/3 -> Mux/3  "ddqd"
  Mux2/1 -> [candlePosition]
  Mux1/1 -> [firstViaPoint]
  Constant4/1 -> Mux1/2  "dqd"
  Constant2/1 -> Mux2/2  "dqd"
  Polynomial Trajectory1/2 -> Mux/2  "dqd"
  [viaPoints] -> Multiport Switch/4
  Selector/1 -> Scope/1, qd/1
  Mux/1 -> [viaPoints]
  Constant5/1 -> Mux2/3  "ddqd"
  [firstViaPoint] -> Multiport Switch/3
  [engageSelectedController] -> Integrator/1
  Constant3/1 -> Mux1/1  "qd"
  Constant6/1 -> Mux1/3  "ddqd"
  Multiport Switch/1 -> Selector2/1, Selector/1, Selector1/1
  [candlePosition] -> Multiport Switch/2
  Selector1/1 -> dqd/1
  Selector2/1 -> ddqd/1

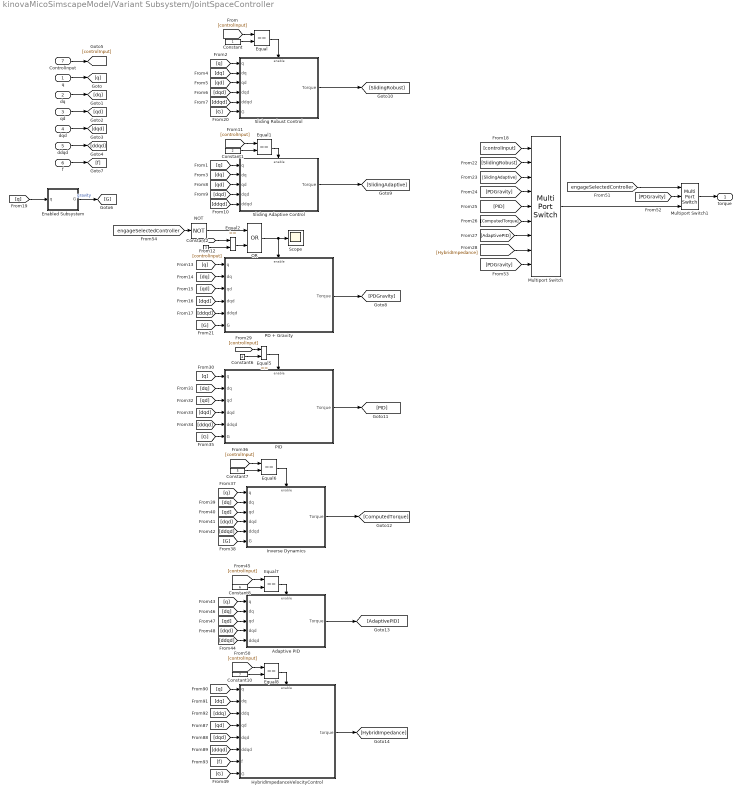
== system kinovaMicoSimscapeModel/Variant Subsystem/JointSpaceController ==
  q : Inport
  dq : Inport  Port=2
  qd : Inport  Port=3
  dqd : Inport  Port=4
  ddqd : Inport  Port=5
  f : Inport  Port=6
  ControlInput : Inport  Port=7
  Adaptive PID : Subsystem  TreatAsAtomicUnit=on
  Constant : Constant
  Constant1 : Constant  Value=2
  Constant10 : Constant  Value=7
  Constant2 : Constant  Value=3
  Constant6 : Constant  Value=4
  Constant7 : Constant  Value=5
  Constant8 : Constant  Value=6
  Enabled Subsystem : Subsystem  TreatAsAtomicUnit=on
  Equal{,1..2,5..8} (7 alike) : RelationalOperator  Operator===  OutDataTypeStr=boolean  RndMeth=Simplest
  HybridImpedanceVelocityControl : Subsystem
  Inverse Dynamics : Subsystem  TreatAsAtomicUnit=on
  Multiport Switch : MultiPortSwitch  Inputs=7  DataPortForDefault=Additional data port  DiagnosticForDefault=None
  Multiport Switch1 : MultiPortSwitch  DataPortOrder=Zero-based contiguous  Inputs=2  zeroidx=on
  NOT : Logic  Operator=NOT  IconShape=distinctive  AllPortsSameDT=off  OutDataTypeStr=boolean
  OR : Logic  Operator=OR  IconShape=distinctive  AllPortsSameDT=off  OutDataTypeStr=boolean
  PD + Gravity : Subsystem  VariantControl=Choice
  PID : Subsystem  VariantControl=Choice
  Scope : Scope
  Sliding Adaptive Control : Subsystem  TreatAsAtomicUnit=on
  Sliding Robust Control : Subsystem  TreatAsAtomicUnit=on
  torque : Outport
  wires:
  [PDGravity] -> Multiport Switch/9
  PID/1(Torque) -> [PID]
  [q] -> Adaptive PID/1(q)
  [q] -> Sliding Adaptive Control/1(q)
  [q] -> Enabled Subsystem/1(q)
  q/1 -> [q]
  [dqd] -> HybridImpedanceVelocityControl/5(dqd)
  Multiport Switch1/1 -> torque/1
  HybridImpedanceVelocityControl/1(torque) -> [HybridImpedance]
  [controlInput] -> Equal7/1
  Sliding Adaptive Control/1(Torque) -> [SlidingAdaptive]
  [dq] -> PID/2(dq)
  [HybridImpedance] -> Multiport Switch/8
  OR/1 -> PD + Gravity/Enable, Scope/1
  ControlInput/1 -> [controlInput]
  [q] -> Sliding Robust Control/1(q)
  [dq] -> Adaptive PID/2(dq)
  [dq] -> Inverse Dynamics/2(dq)
  [controlInput] -> Equal8/1
  [q] -> HybridImpedanceVelocityControl/1(q)
  Constant7/1 -> Equal6/2
  Equal5/1 -> PID/Enable
  [qd] -> PID/3(qd)
  [PID] -> Multiport Switch/5
  [ComputedTorque] -> Multiport Switch/6
  [PDGravity] -> Multiport Switch1/2
  [engageSelectedController] -> NOT/1
  [PDGravity] -> Multiport Switch/4
  [qd] -> HybridImpedanceVelocityControl/4(qd)
  [qd] -> Adaptive PID/3(qd)
  qd/1 -> [qd]
  [dq] -> Sliding Robust Control/2(dq)
  NOT/1 -> OR/1
  Multiport Switch/1 -> Multiport Switch1/3
  Equal2/1 -> OR/2
  Equal8/1 -> HybridImpedanceVelocityControl/Enable
  [engageSelectedController] -> Multiport Switch1/1
  [SlidingAdaptive] -> Multiport Switch/3
  Inverse Dynamics/1(Torque) -> [ComputedTorque]
  PD + Gravity/1(Torque) -> [PDGravity]
  Adaptive PID/1(Torque) -> [AdaptivePID]
  Constant10/1 -> Equal8/2
  [G] -> Sliding Robust Control/6(G)
  Sliding Robust Control/1(Torque) -> [SlidingRobust]
  [G] -> PID/6(G)
  [ddqd] -> Inverse Dynamics/5(ddqd)
  [ddqd] -> HybridImpedanceVelocityControl/6(ddqd)
  [G] -> HybridImpedanceVelocityControl/8(G)
  Constant2/1 -> Equal2/2
  [ddqd] -> Adaptive PID/5(ddqd)
  [q] -> Inverse Dynamics/1(q)
  Equal/1 -> Sliding Robust Control/Enable
  [qd] -> Inverse Dynamics/3(qd)
  [dq] -> HybridImpedanceVelocityControl/2(dq)
  f/1 -> [f]
  Equal1/1 -> Sliding Adaptive Control/Enable
  [G] -> Inverse Dynamics/6(G)
  [ddq] -> HybridImpedanceVelocityControl/3(ddq)
  [dqd] -> Adaptive PID/4(dqd)
  Constant8/1 -> Equal7/2
  [ddqd] -> PD + Gravity/5(ddqd)
  [ddqd] -> Sliding Adaptive Control/5(ddqd)
  [q] -> PD + Gravity/1(q)
  [controlInput] -> Multiport Switch/1
  [qd] -> PD + Gravity/3(qd)
  [controlInput] -> Equal6/1
  Equal7/1 -> Adaptive PID/Enable
  [controlInput] -> Equal5/1
  Equal6/1 -> Inverse Dynamics/Enable
  [q] -> PID/1(q)
  Constant6/1 -> Equal5/2
  Enabled Subsystem/1(G) -> [G]  "gravity"
  [dqd] -> PID/4(dqd)
  [AdaptivePID] -> Multiport Switch/7
  [f] -> HybridImpedanceVelocityControl/7(f)
  [controlInput] -> Equal2/1
  [dq] -> PD + Gravity/2(dq)
  [G] -> PD + Gravity/6(G)
  [ddqd] -> PID/5(ddqd)
  [controlInput] -> Equal1/1
  [qd] -> Sliding Robust Control/3(qd)
  dq/1 -> [dq]
  Constant1/1 -> Equal1/2
  [ddqd] -> Sliding Robust Control/5(ddqd)
  Constant/1 -> Equal/2
  [dqd] -> PD + Gravity/4(dqd)
  [controlInput] -> Equal/1
  [dqd] -> Inverse Dynamics/4(dqd)
  [qd] -> Sliding Adaptive Control/3(qd)
  [dqd] -> Sliding Adaptive Control/4(dqd)
  [dqd] -> Sliding Robust Control/4(dqd)
  [SlidingRobust] -> Multiport Switch/2
  [dq] -> Sliding Adaptive Control/2(dq)
  ddqd/1 -> [ddqd]
  dqd/1 -> [dqd]

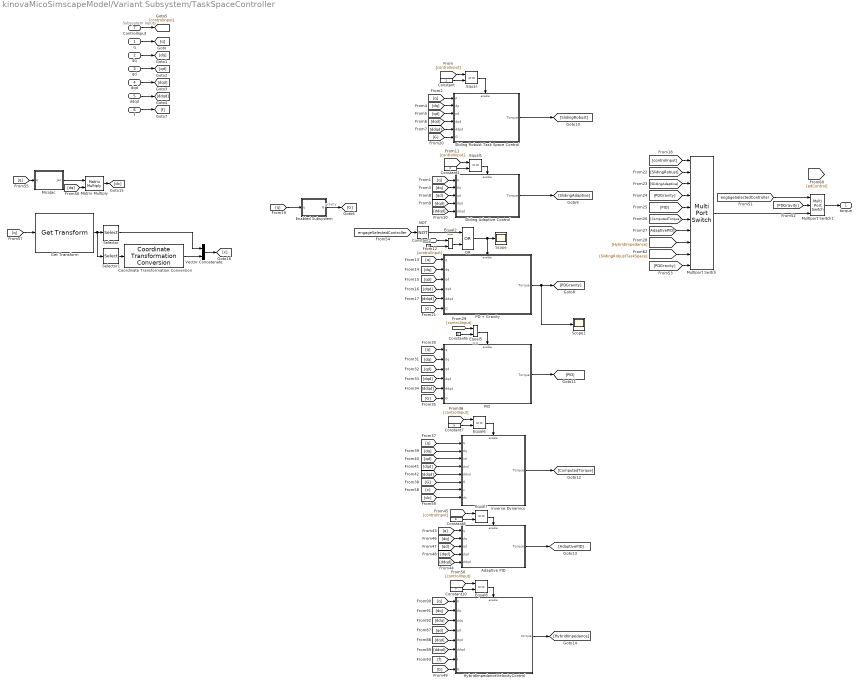
== system kinovaMicoSimscapeModel/Variant Subsystem/TaskSpaceController ==
  note: Subsystem Inputs
  q : Inport
  dq : Inport  Port=2
  qd : Inport  Port=3
  dqd : Inport  Port=4
  ddqd : Inport  Port=5
  f : Inport  Port=6
  ControlInput : Inport  Port=7
  Adaptive PID : Subsystem  TreatAsAtomicUnit=on
  Constant : Constant
  Constant1 : Constant  Value=2
  Constant10 : Constant  Value=7
  Constant2 : Constant  Value=3
  Constant6 : Constant  Value=4
  Constant7 : Constant  Value=5
  Constant8 : Constant  Value=6
  Coordinate Transformation Conversion : robotcorelib/Coordinate Transformation Conversion  InputRepresentation=Rotation Matrix  InputEulerSequence=ZYX  ShowTrVecInputPort=on  OutputRepresentation=Euler Angles  OutputEulerSequence=XYZ  ShowTrVecOutputPort=on  SimulateUsing=Code generation
      settings: SourceProductBaseCode=NV,RO,RR,UV
  Enabled Subsystem : Subsystem  TreatAsAtomicUnit=on
  Equal{,1..2,5..8} (7 alike) : RelationalOperator  Operator===  OutDataTypeStr=boolean  RndMeth=Simplest
  Get Transform : robotmaniplib/Get Transform  RigidBodyTree=mico  SourceBody=EE  TargetBody=base  SimulateUsing=Code generation
  HybridImpedanceVelocityControl : Subsystem
  Inverse Dynamics : Subsystem  TreatAsAtomicUnit=on
  Matrix Multiply : Product  Multiplication=Matrix(*)
  MicoJac : MATLAB Function  TreatAsAtomicUnit=on
  Multiport Switch : MultiPortSwitch  Inputs=8  DataPortForDefault=Additional data port  DiagnosticForDefault=None
  Multiport Switch1 : MultiPortSwitch  DataPortOrder=Zero-based contiguous  Inputs=2  zeroidx=on
  NOT : Logic  Operator=NOT  IconShape=distinctive  AllPortsSameDT=off  OutDataTypeStr=boolean
  OR : Logic  Operator=OR  IconShape=distinctive  AllPortsSameDT=off  OutDataTypeStr=boolean
  PD + Gravity : Subsystem  VariantControl=Choice
  PID : Subsystem  VariantControl=Choice
  Scope : Scope
  Scope1 : Scope
  Selector : Selector  NumberOfDimensions=2  InputPortWidth=3  IndexOptions=Index vector (dialog),Index vector (dialog)  Indices=[1:3],4  OutputSizes=1,1
  Selector1 : Selector  NumberOfDimensions=2  InputPortWidth=3  IndexOptions=Index vector (dialog),Index vector (dialog)  Indices=[1:3],[1:3]  OutputSizes=1,1
  Sliding Adaptive Control : Subsystem  TreatAsAtomicUnit=on
  Sliding Robust Task Space Control : Subsystem  TreatAsAtomicUnit=on
  Vector Concatenate : Concatenate
  torque : Outport
  wires:
  dqd/1 -> [dqd]
  ddqd/1 -> [ddqd]
  [dq] -> Sliding Adaptive Control/2(dq)
  [SlidingRobustTaskSpace] -> Multiport Switch/9
  [SlidingRobust] -> Multiport Switch/2
  [dqd] -> Sliding Adaptive Control/4(dqd)
  [qd] -> Sliding Adaptive Control/3(qd)
  [dqd] -> Inverse Dynamics/4(dxd)
  [controlInput] -> Equal/1
  [dqd] -> PD + Gravity/4(dqd)
  Constant/1 -> Equal/2
  Constant1/1 -> Equal1/2
  dq/1 -> [dq]
  [controlInput] -> Equal1/1
  [ddqd] -> PID/5(ddqd)
  [G] -> PD + Gravity/6(G)
  [dq] -> PD + Gravity/2(dq)
  [controlInput] -> Equal2/1
  [f] -> HybridImpedanceVelocityControl/7(f)
  [AdaptivePID] -> Multiport Switch/7
  [dqd] -> PID/4(dqd)
  Enabled Subsystem/1(G) -> [G]  "gravity"
  Constant6/1 -> Equal5/2
  [q] -> PID/1(q)
  Equal6/1 -> Inverse Dynamics/Enable
  [controlInput] -> Equal5/1
  Equal7/1 -> Adaptive PID/Enable
  [controlInput] -> Equal6/1
  [qd] -> PD + Gravity/3(qd)
  [controlInput] -> Multiport Switch/1
  [q] -> PD + Gravity/1(q)
  [ddqd] -> Sliding Adaptive Control/5(ddqd)
  [qd] -> Sliding Robust Task Space Control/3(pd)
  [ddqd] -> PD + Gravity/5(ddqd)
  Constant8/1 -> Equal7/2
  [dqd] -> Adaptive PID/4(dqd)
  [ddq] -> HybridImpedanceVelocityControl/3(ddq)
  [G] -> Inverse Dynamics/6(G)
  Equal1/1 -> Sliding Adaptive Control/Enable
  f/1 -> [f]
  [dq] -> HybridImpedanceVelocityControl/2(dq)
  [qd] -> Inverse Dynamics/3(xd)
  Equal/1 -> Sliding Robust Task Space Control/Enable
  [q] -> Inverse Dynamics/1(q)
  [ddqd] -> Adaptive PID/5(ddqd)
  Constant2/1 -> Equal2/2
  [G] -> HybridImpedanceVelocityControl/8(G)
  [ddqd] -> HybridImpedanceVelocityControl/6(ddqd)
  [ddqd] -> Inverse Dynamics/5(ddxd)
  [G] -> PID/6(G)
  Sliding Robust Task Space Control/1(Torque) -> [SlidingRobust]
  Constant10/1 -> Equal8/2
  Adaptive PID/1(Torque) -> [AdaptivePID]
  PD + Gravity/1(Torque) -> [PDGravity], Scope1/1
  Inverse Dynamics/1(Torque) -> [ComputedTorque]
  [SlidingAdaptive] -> Multiport Switch/3
  [engageSelectedController] -> Multiport Switch1/1
  Equal8/1 -> HybridImpedanceVelocityControl/Enable
  Equal2/1 -> OR/2
  Multiport Switch/1 -> Multiport Switch1/3
  NOT/1 -> OR/1
  qd/1 -> [qd]
  [qd] -> Adaptive PID/3(qd)
  [qd] -> HybridImpedanceVelocityControl/4(qd)
  [PDGravity] -> Multiport Switch/4
  [engageSelectedController] -> NOT/1
  [PDGravity] -> Multiport Switch1/2
  [ComputedTorque] -> Multiport Switch/6
  [PID] -> Multiport Switch/5
  [qd] -> PID/3(qd)
  [G] -> Sliding Robust Task Space Control/6(G)
  Equal5/1 -> PID/Enable
  Constant7/1 -> Equal6/2
  [q] -> HybridImpedanceVelocityControl/1(q)
  [controlInput] -> Equal8/1
  [dq] -> Inverse Dynamics/2(dq)
  [dq] -> Adaptive PID/2(dq)
  [dqd] -> Sliding Robust Task Space Control/4(dpd)
  ControlInput/1 -> [controlInput]
  OR/1 -> Scope/1, PD + Gravity/Enable
  [HybridImpedance] -> Multiport Switch/8
  [dq] -> PID/2(dq)
  Sliding Adaptive Control/1(Torque) -> [SlidingAdaptive]
  [controlInput] -> Equal7/1
  HybridImpedanceVelocityControl/1(torque) -> [HybridImpedance]
  Multiport Switch1/1 -> torque/1
  [dqd] -> HybridImpedanceVelocityControl/5(dqd)
  q/1 -> [q]
  [q] -> Sliding Robust Task Space Control/1(p)
  [q] -> Enabled Subsystem/1(q)
  [q] -> Sliding Adaptive Control/1(q)
  [q] -> Adaptive PID/1(q)
  [dq] -> Sliding Robust Task Space Control/2(dp)
  PID/1(Torque) -> [PID]
  [ddqd] -> Sliding Robust Task Space Control/5(ddpd)
  [PDGravity] -> Multiport Switch/10
  [q] -> MicoJac/1(q)
  MicoJac/1(Jac) -> Matrix Multiply/1
  [dq] -> Matrix Multiply/2
  Matrix Multiply/1 -> [dx]
  [q] -> Get Transform/1
  Get Transform/1 -> Selector1/1, Selector/1
  [x] -> Inverse Dynamics/7(x)
  [dx] -> Inverse Dynamics/8(dx)
  Selector1/1 -> Coordinate Transformation Conversion/1
  Selector/1 -> Vector Concatenate/1
  Vector Concatenate/1 -> [x]
  Coordinate Transformation Conversion/1 -> Vector Concatenate/2

== system kinovaMicoSimscapeModel/StateErrorNorm/JointSpaceError/Compute dqError ==
  dqd : Inport
  dq : Inport  Port=2
  Dot Product : DotProduct  InputSameDT=on  OutDataTypeStr=Inherit: Inherit via internal rule
  Sqrt : Sqrt  SaturateOnIntegerOverflow=on
  Subsystem : Subsystem  Commented=on
  Sum : Sum  Inputs=|+-
  dq_error : Outport
  wires:
  Sqrt/1 -> dq_error/1
  dq/1 -> Sum/2
  dqd/1 -> Sum/1
  Dot Product/1 -> Sqrt/1
  Sum/1 -> Dot Product/1, Dot Product/2

== system kinovaMicoSimscapeModel/StateErrorNorm/JointSpaceError/Compute qError ==
  qd : Inport
  q : Inport  Port=2
  Dot Product : DotProduct  InputSameDT=on  OutDataTypeStr=Inherit: Inherit via internal rule
  Sqrt : Sqrt  SaturateOnIntegerOverflow=on
  Subsystem : Subsystem  Commented=on
  Sum : Sum  Inputs=|+-
  q_error : Outport
  wires:
  Sum/1 -> Dot Product/2, Dot Product/1
  Dot Product/1 -> Sqrt/1
  qd/1 -> Sum/1
  q/1 -> Sum/2
  Sqrt/1 -> q_error/1
